simulink library "library"  (R2018b)
settings: Solver=VariableStepAuto  StartTime=0.0  StopTime=10.0  RelTol=1e-3
libraries: visionfilter x2, visionstatistics x1
settings Model: Creator=dgaiero  LastModifiedBy=dgaiero

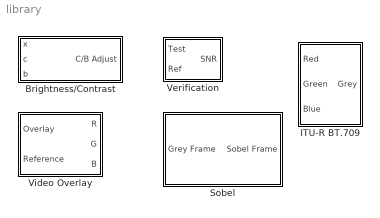
== system library ==
  Brightness/Contrast : Subsystem
  ITU-R BT.709 : Subsystem
  Sobel : Subsystem
  Verification : Subsystem
  Video Overlay : Subsystem  mask{rChannelThreshold=0.7, gChannelThreshold=0.7, bChannelThreshold=0.7}
      mask prompts: rChannelThreshold "Red Channel Threshold"; gChannelThreshold "Green Channel Threshold"; bChannelThreshold "Blue Channel Threshold"
      mask TypeOptions rChannelThreshold: Switch - R/Threshold
      mask TypeOptions gChannelThreshold: Switch - G/Threshold
      mask TypeOptions bChannelThreshold: Switch - B/Threshold

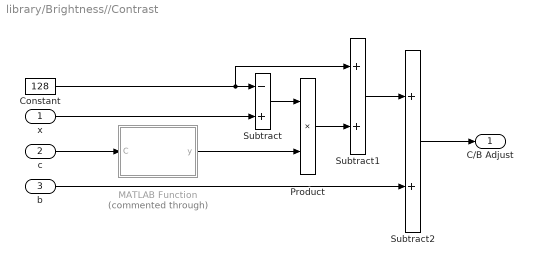
== system library/Brightness//Contrast ==
  x : Inport
  c : Inport  Port=2
  b : Inport  Port=3
  Constant : Constant  Value=128  SampleTime=-1
  MATLAB Function : MATLAB Function  Commented=through  TreatAsAtomicUnit=on
  Product : Product
  Subtract : Sum  Inputs=-+
  Subtract1 : Sum
  Subtract2 : Sum
  C/B Adjust : Outport
  wires:
  Constant/1 -> Subtract1/1, Subtract/1
  x/1 -> Subtract/2
  Subtract/1 -> Product/1
  c/1 -> MATLAB Function/1(C)
  Product/1 -> Subtract1/2
  Subtract1/1 -> Subtract2/1
  b/1 -> Subtract2/2
  Subtract2/1 -> C/B Adjust/1
  MATLAB Function/1(y) -> Product/2

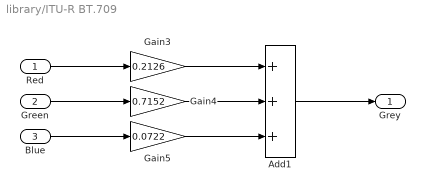
== system library/ITU-R BT.709 ==
  Red : Inport
  Green : Inport  Port=2
  Blue : Inport  Port=3
  Add1 : Sum  Inputs=3
  Gain3 : Gain  Gain=0.2126
  Gain4 : Gain  Gain=0.7152
  Gain5 : Gain  Gain=0.0722
  Grey : Outport
  wires:
  Gain3/1 -> Add1/1
  Gain4/1 -> Add1/2
  Gain5/1 -> Add1/3
  Add1/1 -> Grey/1
  Red/1 -> Gain3/1
  Green/1 -> Gain4/1
  Blue/1 -> Gain5/1

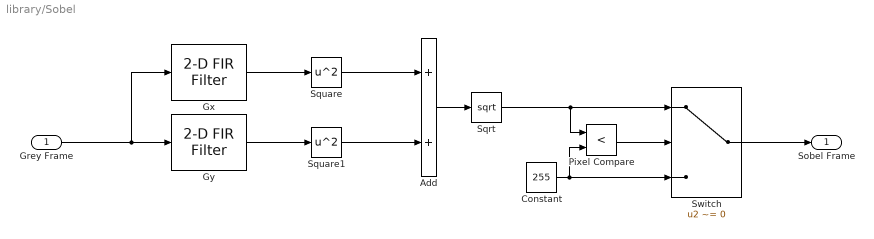
== system library/Sobel ==
  Grey Frame : Inport
  Add : Sum
  Constant : Constant  Value=255
  Gx : visionfilter/2-D FIR Filter  separable=off  filtSrc=Specify via dialog  filterMtrx=[-1 0 1;-2 0 2; -1 0 1]  verticalFilter=[4 0]  horizontalFilter=[4 0]  outSize=Same as input port I  padType=Replicate  padSrc=Specify via dialog  padVal=0  method=Convolution  firstCoeffMode=Specify word length  firstCoeffWordLength=16  firstCoeffFracLength=14  firstCoeffSignedness=Signed  firstCoeffDataTypeStr=fixdt(1,16)  firstCoeffLastDataTypeStr=fixdt(1,16)  firstCoeffMin=[]  firstCoeffMax=[]  outputSignedness=Auto  outputMin=[]  outputMax=[]  accumDataTypeStr=Inherit: Same as product output  accumLastDataTypeStr=Inherit: Same as product output  prodOutputMode=Binary point scaling  prodOutputWordLength=32  prodOutputFracLength=10  prodOutputDataTypeStr=fixdt([],32,10)  prodOutputLastDataTypeStr=fixdt([],32,10)  roundingMode=Floor  overflowMode=off
      settings: SourceProductName=Computer Vision System Toolbox  SourceProductBaseCode=VP
  Gy : visionfilter/2-D FIR Filter  separable=off  filtSrc=Specify via dialog  filterMtrx=[+1 +2 +1;0 0 0;-1 -2 -1]  verticalFilter=[4 0]  horizontalFilter=[4 0]  outSize=Same as input port I  padType=Replicate  padSrc=Specify via dialog  padVal=0  method=Convolution  firstCoeffMode=Specify word length  firstCoeffWordLength=16  firstCoeffFracLength=14  firstCoeffSignedness=Signed  firstCoeffDataTypeStr=fixdt(1,16)  firstCoeffLastDataTypeStr=fixdt(1,16)  firstCoeffMin=[]  firstCoeffMax=[]  outputSignedness=Auto  outputMin=[]  outputMax=[]  accumDataTypeStr=Inherit: Same as product output  accumLastDataTypeStr=Inherit: Same as product output  prodOutputMode=Binary point scaling  prodOutputWordLength=32  prodOutputFracLength=10  prodOutputDataTypeStr=fixdt([],32,10)  prodOutputLastDataTypeStr=fixdt([],32,10)  roundingMode=Floor  overflowMode=off
      settings: SourceProductName=Computer Vision System Toolbox  SourceProductBaseCode=VP
  Pixel Compare : RelationalOperator  Operator=<  OutDataTypeStr=boolean  RndMeth=Simplest
  Sqrt : Sqrt  IntermediateResultsDataTypeStr=double  SaturateOnIntegerOverflow=on
  Square : Math  Operator=square  RndMeth=Zero  SaturateOnIntegerOverflow=on
  Square1 : Math  Operator=square  RndMeth=Zero  SaturateOnIntegerOverflow=on
  Switch : Switch  Criteria=u2 ~= 0  Threshold=255
  Sobel Frame : Outport
  wires:
  Pixel Compare/1 -> Switch/2
  Constant/1 -> Switch/3, Pixel Compare/2
  Square1/1 -> Add/2
  Grey Frame/1 -> Gx/1, Gy/1
  Gx/1 -> Square/1
  Switch/1 -> Sobel Frame/1
  Gy/1 -> Square1/1
  Add/1 -> Sqrt/1
  Square/1 -> Add/1
  Sqrt/1 -> Switch/1, Pixel Compare/1

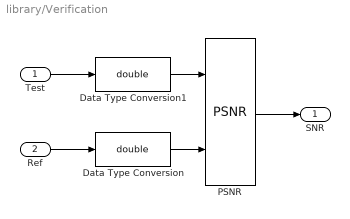
== system library/Verification ==
  Test : Inport
  Ref : Inport  Port=2
  Data Type Conversion : DataTypeConversion  OutDataTypeStr=double
  Data Type Conversion1 : DataTypeConversion  OutDataTypeStr=double
  PSNR : visionstatistics/PSNR
      settings: SourceProductName=Computer Vision System Toolbox  SourceProductBaseCode=VP
  SNR : Outport
  wires:
  Data Type Conversion/1 -> PSNR/2
  PSNR/1 -> SNR/1
  Test/1 -> Data Type Conversion1/1
  Ref/1 -> Data Type Conversion/1
  Data Type Conversion1/1 -> PSNR/1

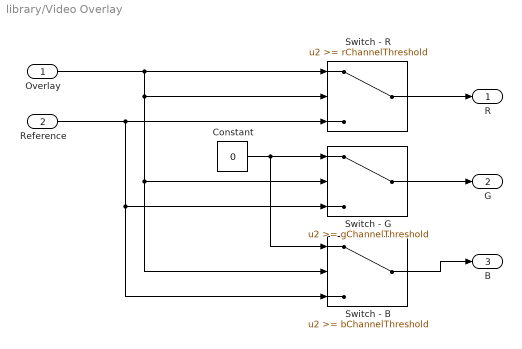
== system library/Video Overlay ==
  Overlay : Inport
  Reference : Inport  Port=2
  Constant : Constant  Value=0  SampleTime=-1
  Switch - B : Switch  Threshold=bChannelThreshold
  Switch - G : Switch  Threshold=gChannelThreshold
  Switch - R : Switch  Threshold=rChannelThreshold
  R : Outport
  G : Outport  Port=2
  B : Outport  Port=3
  wires:
  Switch - G/1 -> G/1
  Switch - B/1 -> B/1
  Reference/1 -> Switch - R/3, Switch - G/3, Switch - B/3
  Switch - R/1 -> R/1
  Constant/1 -> Switch - G/1, Switch - B/1
  Overlay/1 -> Switch - R/1, Switch - R/2, Switch - G/2, Switch - B/2

== matlab function library/Brightness//Contrast/MATLAB Function ==
  data: C input; y output
function y = F(C)
y=(259*(C+255))/(255*(259-C));
